simulink model "complete_plant"  (R2022a)
settings: Solver=ode45  StartTime=0.0  StopTime=15  RelTol=1e-3
values from neighbouring files (symbols this model uses):
  a = Simulink.Parameter(1.14)    [startup.m]
  A1 = Simulink.Parameter(39.8344)    [startup.m]
  A2 = Simulink.Parameter(813.0780)    [startup.m]
  absolute_batter_power_limit = Simulink.Parameter(75000)    [startup.m]
  b = Simulink.Parameter(-0.03291)    [startup.m]
  B1 = Simulink.Parameter(0.000001287)    [startup.m]
  B2 = Simulink.Parameter(-0.002325)    [startup.m]
  B3 = Simulink.Parameter(3.797)    [startup.m]
  brake_start = 30    [startup.m]
  c = Simulink.Parameter(-1.14)    [startup.m]
  C1 = Simulink.Parameter(-0.000000002541)    [startup.m]
  C2 = Simulink.Parameter(0.000005279)    [startup.m]
  C3 = Simulink.Parameter(-0.003943)    [startup.m]
  C4 = Simulink.Parameter(3.634)    [startup.m]
  C_param = Simulink.Parameter([0 13757.41 21278.97 26666.02 30253.47 30313.18 30313.18])    [startup.m]
  d = Simulink.Parameter(-1.027)    [startup.m]
  deadband_velocity = Simulink.Parameter(0.5)    [startup.m]
  distance_traveled = 75    [startup.m]
  dTx = 0.01    [startup.m]
  FZ_C = Simulink.Parameter([0 204.13 427.04 668.1 895.72 1124.40 1324.40])    [startup.m]
  gr = Simulink.Parameter([6.63043, 6.63043, 8, 8])    [startup.m]
  I = 15    [startup.m]
  inch2mm = Simulink.Parameter(25.4)    [startup.m]
  J_z = Simulink.Parameter(75)    [startup.m]
  k_limit = Simulink.Parameter(3.461)    [startup.m]
  Ku = Simulink.Parameter(0.24 / g.Value)    [startup.m]
  l = Simulink.Parameter([0.7922471, 0.7828529])    [startup.m]
  max_motor_temp = 75    [startup.m]
  max_yaw_field = Simulink.Parameter([1.34 1.34 1.34 1.66 1.14 1.24 0.754 0.849 0.85 0.85])    [startup.m]
  min_velocity_regen = Simulink.Parameter(1.4)    [startup.m]
  motor_efficiency = Simulink.Parameter([0.9, 0.9, 0.9, 0.9])    [startup.m]
  motor_limit_torque = Simulink.Parameter([-25, 25])    [startup.m]
  mu_factor = Simulink.Parameter(0.7)    [startup.m]
  P = 1    [startup.m]
  power_loss_limit = Simulink.Parameter([0, 0, 1800, 1800])    [startup.m]
  RE = Simulink.Parameter(0.2228169203)    [startup.m]
  s = Simulink.Parameter([0.647895, 0.62102])    [startup.m]
  S1 = Simulink.Parameter(7 * (10^(-5)))    [startup.m]
  S2 = Simulink.Parameter(-0.0038)    [startup.m]
  S3 = Simulink.Parameter(0.6535)    [startup.m]
  S4 = Simulink.Parameter(0.1061)    [startup.m]
  steer_slope = Simulink.Parameter(0.0111)    [startup.m]
  T = 0    [startup.m]
  T2F = Simulink.Parameter(single([4.385 4.385 4.385 4.385]))    [startup.m]
  target_velocity = 35    [startup.m]
  tau = Simulink.Parameter(0)    [startup.m]
  time_delay = 0.022    [startup.m]
  V_target = Simulink.Parameter([0 3 6 9 12 15 18 21 25 31])    [startup.m]
  Vth = Simulink.Parameter(2)    [startup.m]
undefined symbols (not defined in the file or in its folder): Ag, brake_pressure, DiscIntNeverNeededParam, driver_input, efficiency_grid, FZ, max_rpm, max_torque, motor_temp, omega, power_limits, power_loss_grid, psi, rdot, rpm_sweep, shock_displacement, shock_velocity, steering_angle, torque_sweep, Vg, y, yaw
libraries: fl_lib x20, nesl_utility x12, sdl_lib x4, slpidlib x2, vehdynlibtire x2, autolibdatasheetbattery x1, autolibmappedmotor x1, autolibshared x1, vehdynlibviscommon x1
(part 4 of 4)

== matlab function complete_plant/Electronics/Torque Vectoring FPGA/Optimization  ==
  settings: updateMethod=DISCRETE
  data: previous_Tx input size=[1 4]; Tx_actual output double size=[1 4]; driver_input input size=1; velocity input size=[1 2]; min_velocity_regen parameter size=1; bigM_flag output size=1; typed output size=1; lb input size=[1 4]; ub input size=[1 4]; A input size=[1 4]; b input size=1; Aeq input size=[1 4]; beq input size=1; T2F parameter size=[1 4]; gr parameter size=[1 4]; lb_adjust output; ub_adjust output; target_velocity parameter; dTx parameter; lb_plus output; ub_neg output
function [Tx_actual, bigM_flag, typed, lb_adjust, ub_adjust, lb_plus, ub_neg] = optimization(previous_Tx, driver_input, velocity, min_velocity_regen, lb, ub, A, b, Aeq, beq, T2F, gr, target_velocity, dTx)
%% LP_calc Computation
% Developer(s):    David Farell
%                  Demetrius Gulewicz
%                  Elliot Stockwell
%                  Tao Sun
%
% Developed for: Purdue Electric Racing
% Date:          12/25/2021
%
% Description: This function primarily computes the desired torque
%              distribution after constructing an optimization statement.
%
%
%% Pass Through Signals
% omega_m - Motor Shaft Angular Velocity [rad/s][1x4]
%
%
%% Input Only
% prev_torque - Torque Requested To Motor In Previous Time Step [Nm][4x1]
% driver_input - Proportion of total available power to use [Unitless][1x1]
% T2F - Convert Torque At The Motor Shaft to Force At The Tire [1/m][1x4]
% power_limit_battery - Max & Min Total Battery Power Output [W][1x2]
% FY - Tires Forces y Direction, Tire fixed coordinates [N][1x4]
% x - Equivalent Distances That FX Acts From CoG [m][1x4]
% y - Equivalent Distances That FY Acts From CoG [m][1x4]
% slip_limit - Max Torque Before Tire Slips [Nm][1x4]
% torque_limit_motor - Max Torque Motor Can Output [Nm][1x4]
% tau_limit_upper - Max Torque Motor Is Allowed To Change To [Nm][1x4]
% tau_limit_lower - Min Torque Motor Is Allowed To Change To [Nm][1x4]
% PID - Desired Yaw Acceleration [rad/s^2][1x1]
%
%
%% Output Only
% Tx - Torque Request To Motors [Nm][4x1]
% lb - Min Torque Request [Nm][1x4]
% ub - Max Torque Request [Nm][1x4]
% Aeq - Moment About CoG, Optimization Variable [rad/s^2][1x1]
% beq - Moment About CoG, Yaw Acceleration & Other Foces [rad/s^2][1x1]
% A - Power Consumed, Optimization Variable [W][1x1]
% b - Power Consumed, Driver Input [W][1x1]
% M_max - Max & Min Yaw Acceleration Achievable With lb & ub [rad/s^2][1x2]
% Power - Total Estimated Power Consumed by the 4 Motors
% TR - The Estimated Yaw Acceleration from the Vehicle
%
%
%% Constants
% global J_z; % Polar Moment Of Inertia [kg m^2][1x1]
% global motor_efficiency; % Motor efficiency [Unitless][1x4]
% global motor_limit_torque; % Minimum & Max Torque Request From Motor [Nm][1x2]
% global min_speed_regen; % Min Motor Shaft Speed For Regen Braking [rad/s][1x1]
% T2F - Convert Torque At The Motor Shaft to Force At The Tire [1/m][1x4]


%% Temporary
Vg = norm(velocity);


%% Detect Potential Zero Crossing, Determine Augmented lb and ub
lb_plus = lb;
ub_neg = ub;
zero_crossing = 0;
crossing_locations = [0 0 0 0];
yaw_error_limit = 0.2;

for i = 1:4
    if lb_plus(i) <= 0 && ub_neg(i) >= 0
        zero_crossing = 1;
        crossing_locations(i) = i;
        
        if previous_Tx(i) >= 0
            lb_plus(i) = dTx / 2;
            ub_neg(i) = ub(i);
        elseif previous_Tx(i) < 0
            lb_plus(i) = lb(i);
            ub_neg(i) = -dTx / 2;          
        end
%     elseif abs(ub(i) - lb(i)) < 0.5
%         ub_neg(i) = -0.1; 
%         lb_plus(i) = -10;
%         lb(i) = -0.002;
%         ub(i) = 0.002;
    end
end

signs = sign(lb_plus);

             
%% Optimization
Tx = single([0 0 0 0]);
bigM_flag = single(0);
typed = 0;
ub_adjust = [0 0 0 0];
lb_adjust = [0 0 0 0];
signs_adjust = [0 0 0 0];

if driver_input < 0
    T2F_aug = -T2F .* gr;
    A = -A;
else
    T2F_aug = T2F .* gr;
end

% if Vg < min_velocity_regen
%     signs_use = abs(signs);
% elseif (target_velocity - velocity(1)) < 1
%     signs_use = abs(signs);
% else
%     signs_use = signs;
% end

if ~(Vg < min_velocity_regen && driver_input < 0)
    if zero_crossing
            % Zero Crossing Primary Optimization
            [Tx21, Tx22, Tx23, Tx24, bigM_flag2] = call_bigM_C(T2F_aug, b, A, beq, Aeq, lb_plus, ub_neg, signs, yaw_error_limit);           
            Tx2 = double([Tx21, Tx22, Tx23, Tx24]);
            
            for i = 1:4
                if abs(Tx2(i)) <= dTx && abs(Tx2(i)) >= dTx/2 && crossing_locations(i) > 0
                    if signs(i) > 0
                        lb_adjust(i) = lb(i);
                        ub_adjust(i) = -lb_plus(i);
                    else
                        lb_adjust(i) = -ub_neg(i);
                        ub_adjust(i) = ub(i);  
                    end
                elseif crossing_locations(i) > 0
                    lb_adjust(i) = lb_plus(i);
                    ub_adjust(i) = ub_neg(i);
                else
                    lb_adjust(i) = lb(i);
                    ub_adjust(i) = ub(i);
                end
            end
            
            signs_adjust = sign(lb_adjust);

%             if Vg < min_velocity_regen
%                 signs_adjust_use = abs(signs_adjust);
%             elseif  (target_velocity - velocity(1)) < 1
%                 signs_adjust_use = abs(signs_adjust);
%             else
%                 signs_adjust_use = signs_adjust;
%             end

            [Tx31, Tx32, Tx33, Tx34, bigM_flag3] = call_bigM_C(T2F_aug, b, A, beq, Aeq, lb_adjust, ub_adjust, signs_adjust, yaw_error_limit);
            Tx3 = double([Tx31, Tx32, Tx33, Tx34]);
            
            % Zero Crossing Secondary Optimization
%             [Tx5, bigM_flag5] = call_bigM_alt(b, A, beq, Aeq, lb, ub_neg);
%             
%             for i = 1:4
%                 if abs(Tx5(i)) < 0.002 && abs(Tx5(i)) >= 0.001 && crossing_locations(i) > 0
%                     if signs(i) > 0
%                         lb_adjust(i) = lb(i);
%                         ub_adjust(i) = -lb_plus(i);
%                     else
%                         lb_adjust(i) = -ub_neg(i);
%                         ub_adjust(i) = ub(i);  
%                     end
%                 elseif crossing_locations(i) > 0
%                     lb_adjust(i) = lb_plus(i);
%                     ub_adjust(i) = ub_neg(i);
%                 else
%                     lb_adjust(i) = lb(i);
%                     ub_adjust(i) = ub(i);
%                 end
%             end
%             
%             [Tx6, bigM_flag6] = call_bigM_alt(b, A, beq, Aeq, lb_adjust, ub_adjust);
            
            % Optimization Selection
            if bigM_flag3 == 1 || bigM_flag3 == 3
                Tx = single(Tx3);
                typed = 3;
                bigM_flag = single(bigM_flag3);
            else
                Tx = single([0 0 0 0]);
                typed = 6;
                bigM_flag = single(bigM_flag3);
            end
    else    
        % No Zero Crossing
        [Tx11, Tx12, Tx13, Tx14, bigM_flag1] = call_bigM_C(T2F_aug, b, A, beq, Aeq, lb, ub, signs, 0.05);
        Tx1 = [Tx11, Tx12, Tx13, Tx14];
%         [Tx4, bigM_flag4] = call_bigM_alt(b, A, beq, Aeq, lb, ub);
        
        % Optimization Selection
        if bigM_flag1 == 3 || bigM_flag1 == 1
            Tx = single(Tx1);
            typed = 1;
            bigM_flag = single(bigM_flag1);
        else
            Tx = single(previous_Tx);
            typed = 4;
            bigM_flag = single(bigM_flag1);
        end   
    end
else
    typed = 7;
    bigM_flag = single(3);
end

Tx_actual = double(Tx);


% Torque Deadband for small input / discritization issues
for i = 1:4
    if abs(Tx_actual(i)) < 2*dTx
        Tx_actual(i) = 0;
    end
end


%% Simplified Control Scheme
% Tx_actual = driver_input .* [25 25 25 25];


end

== matlab function complete_plant/Driver/Longitudinal Control/MATLAB Function ==
  data: driver_input input; brake_pressure output
function brake_pressure = fcn(driver_input)

    if driver_input < 0
        brake_pressure = [1 1 1 1] .* driver_input .* 10;
    else
        brake_pressure = [0 0 0 0];
    end

end

== matlab function complete_plant/Vehicle Model/Tires/MATLAB Function1 ==
  data: yaw input; V_tx output size=[1 4]; Vg input; steering_angles input; s parameter; l parameter; V_ty output size=[1 4]
function [V_tx, V_ty] = get_tire_velocities(yaw, Vg, steering_angles, s, l)
coder.extrinsic('round')

V_fl = Vg + (yaw .* [s(1) l(1)]);
V_fr = Vg + (yaw .* [-s(1) l(1)]);
V_rl = Vg + (yaw .* [s(2) -l(2)]);
V_rr = Vg + (yaw .* [-s(2) -l(2)]);

V_x = [V_fl(1) V_fr(1) V_rl(1) V_rr(1)];
V_y = [V_fl(2) V_fr(2) V_rl(2) V_rr(2)];

steering_angles = -steering_angles;

input = [V_y; V_x];

transform_matrix_FL = [cos(steering_angles(1)) sin(steering_angles(1)); -sin(steering_angles(1)) cos(steering_angles(1))];
transform_matrix_FR = [cos(steering_angles(2)) sin(steering_angles(2)); -sin(steering_angles(2)) cos(steering_angles(2))];
transform_matrix_RL = [cos(0) sin(0); -sin(0) cos(0)];
transform_matrix_RR = [cos(0) sin(0); -sin(0) cos(0)];

V_FL = transform_matrix_FL * input(:, 1);
V_FR = transform_matrix_FR * input(:, 2);
V_RL = transform_matrix_RL * input(:, 3);
V_RR = transform_matrix_RR * input(:, 4);

% V_tx = zeros(1, 4);
% V_ty = zeros(1, 4);
% 
% V_tx = round([V_FL(2) V_FR(2) V_RL(2) V_RR(2)], 2);
% V_ty = round([-V_FL(1) -V_FR(1) -V_RL(1) -V_RR(1)], 2);

V_tx = [V_FL(2) V_FR(2) V_RL(2) V_RR(2)];
V_ty = [-V_FL(1) -V_FR(1) -V_RL(1) -V_RR(1)];

== matlab function complete_plant/Sensors/MATLAB Function ==
  data: driver_input input; driver_input output
function driver_input = fcn(driver_input)
if driver_input < 0.01 && driver_input > -0.01
    driver_input = 0;
end

== matlab function complete_plant/Electronics/Torque Vectoring Micro Controller/Tire Model ==
  data: FZ input size=[1 4]; Fx_max output size=[1 4]; Vg input size=[1 2]; yaw input size=1; omega input size=[1 4]; steering input size=[1 3]; FY output size=[1 4]; s parameter size=[1 2]; l parameter size=[1 2]; RE parameter size=1; A1 parameter size=1; A2 parameter size=1; B1 parameter size=1; B2 parameter size=1; B3 parameter size=1; C1 parameter size=1; C2 parameter size=1; C3 parameter size=1; C4 parameter size=1; FZ_C parameter size=[1 7]; C_param parameter size=[1 7]; a parameter size=1; b parameter size=1; c parameter size=1; d parameter size=1; k_limit parameter size=1; mu_factor parameter size=1; FX output; Vth parameter
function [Fx_max, FY, FX] =  tire_model( FZ, Vg, yaw, omega, steering, s, l, RE, A1, A2, B1, B2, B3, C1, C2, C3, C4, FZ_C, C_param, a, b, c, d, k_limit, mu_factor, Vth)
%% Compute Steering Angles
acker_steer_angles = [steering(2) steering(3)];
Vx = Vg(1);
Vy = Vg(2);

%% Compute Tire Slip
% Velocity at each Tire
V_fl = Vg + (yaw .* [s(1) l(1)]);
V_fr = Vg + (yaw .* [-s(1) l(1)]);
V_rl = Vg + (yaw .* [s(2) -l(2)]);
V_rr = Vg + (yaw .* [-s(2) -l(2)]);

rotation_matrix_FL = [cos(acker_steer_angles(1)) sin(acker_steer_angles(1)); -sin(acker_steer_angles(1)) cos(acker_steer_angles(1))];
rotation_matrix_FR = [cos(acker_steer_angles(2)) sin(acker_steer_angles(2)); -sin(acker_steer_angles(2)) cos(acker_steer_angles(2))];

V_fl = rotation_matrix_FL * [V_fl(2); V_fl(1)];
V_fr = rotation_matrix_FR * [V_fr(2); V_fr(1)];

% Individual slip angles, it blows up at low velocity
if abs(Vg(1)) > Vth
    SA_fl = -atan2(Vy + (l(1)*yaw), Vx + (s(1)*yaw)) + acker_steer_angles(1);
    SA_fr = -atan2(Vy + (l(1)*yaw), Vx - (s(1)*yaw)) + acker_steer_angles(2);
    SA_rl = -atan2(Vy - (l(2)*yaw), Vx + (s(2)*yaw));
    SA_rr = -atan2(Vy - (l(2)*yaw), Vx - (s(2)*yaw));
else
    SA_fl = 0;
    SA_fr = 0;
    SA_rl = 0;
    SA_rr = 0;
end

SA = [SA_fl SA_fr SA_rl SA_rr];

% Compute Slip Ratio
if Vg(1) > Vth
    SL_fl = ((RE * omega(1)) / (V_fl(2) * cos(SA_fl))) - 1;
    SL_fr = ((RE * omega(2)) / (V_fr(2) * cos(SA_fr))) - 1;
    SL_rl = ((RE * omega(3)) / (V_rl(1) * cos(SA_rl))) - 1;
    SL_rr = ((RE * omega(4)) / (V_rr(1) * cos(SA_rr))) - 1;
else
    SL_fl = ((RE * omega(1)) - V_fl(2)) / (Vth + (V_fl(2)^2 / Vth));
    SL_fr = ((RE * omega(2)) - V_fr(2)) / (Vth + (V_fr(2)^2 / Vth));
    SL_rl = ((RE * omega(3)) - V_rl(1)) / (Vth + (V_rl(1)^2 / Vth));
    SL_rr = ((RE * omega(4)) - V_rr(1)) / (Vth + (V_rr(1)^2 / Vth));
end

SL = [SL_fl SL_fr SL_rl SL_rr];

%% Non Dimensional Tire Model
% Basic Coefficients
kx = (A1 .* (FZ)) + A2;
C = pchip(FZ_C, C_param, abs(FZ));
mu_x = ((B1 .* (FZ.^2)) + (B2 .* (FZ)) + B3);
mu_y = ((C1 .* (FZ.^3)) + (C2 .* (FZ.^2)) + (C3 .* (FZ)) + C4);

% Normalized Slip Ratio, Slip Angle
s_bar = (kx .* SL) ./ (mu_x .* FZ);

% C is a function of FZ, but it is not an analytical expression
a_bar = (C .* tan(SA)) ./ (mu_y .* FZ);

% Combined Slip Model Parameters
n0 = (C .* mu_x) ./ (kx .* mu_y);
k = sqrt(s_bar.^2 + a_bar.^2);
n = [1 1 1 1];

for i = 1:4
    if abs(k(i)) <= (2*pi)
       n = (0.5 .* (1 + n0)) - (0.5 .* cos(k/2) .* (1 - n0));
    end
end

% Compute R, the bridge between tire slip and tire forces
R = (a .* exp(b .* k)) + (c .* exp(d .* k));

% Compute FX & FY
if (sum(SL==0) + sum(SA==0)) == 8
    FX = [0 0 0 0];
    FY = [0 0 0 0];
else
    FX = (mu_x .* FZ .* R .* SL) ./ (sqrt(SL.^2 + ((n.^2) .* (tan(SA)).^2)));
    FY = (n .* R .* tan(SA) .* mu_y .* FZ) ./ (sqrt(SL.^2 + ((n.^2) .* (tan(SA)).^2)));
end

%% Max Longitudinal Force
% Constant during runtime
R_max = [1 1 1 1] .* (a .* exp(b .* k_limit)) + (c .* exp(d .* k_limit));
n_max = [1 1 1 1];

if abs(k(i)) <= (2*pi)
   n_max = [1 1 1 1] .* (0.5 .* (1 + n0)) - (0.5 .* cos(k_limit/2) .* (1 - n0));
end

s_bar_max = [0 0 0 0];

for i = 1:4
    if k_limit > abs(a_bar(i))
        s_bar_max(i) = sqrt(k_limit^2 - a_bar(i)^2);
    end
end

SL_max = (s_bar_max .* mu_x .* FZ) ./ (kx);

Fx_max = (mu_x .* FZ .* R_max .* SL_max) ./ (sqrt(SL_max.^2 + ((n_max.^2) .* (tan(SA)).^2)));

if sum(abs(SL(3:4)) > 0.3) > 0
   Fx_max(3:4) = [500 500];
end

if sum(abs(SL(1:2)) > 0.3) > 0
   Fx_max(1:2) = [500 500];
end

%% Compute Corrected FX & FY
FY = FY .* mu_factor;
FX = FX .* mu_factor;
Fx_max = Fx_max .* mu_factor;
end

== matlab function complete_plant/Electronics/Torque Vectoring Micro Controller/Brake Model ==
  data: brake_pressure input size=[1 4]; T_brake output size=[1 4]; V input size=[1 2]; brakecoeff parameter size=[1 4]
function T_brake = brake_model(brake_pressure, V, brakecoeff)
%% Inputs
% brake_pressure_front     [MPa]
% brake_pressure_rear      [MPa]
% omega_wheel_RL           [rad/s]

%% Outputs
% T_Brake                  [Nm][1x4]
%    T_Brake_FL
%    T_Brake_FR
%    T_Brake_RL
%    T_Brake_RR


%% Compute
T_brake = zeros(1, 4);

if abs(V(1)) > 5
   T_brake = brakecoeff .* sign(V(1)) .* brake_pressure;
end

end
